simulink model "simulacion_sin_f"  (R2021a)
settings: Solver=VariableStepAuto  StartTime=0.0  StopTime=10.0  RelTol=1e-3
libraries: simulink x1
settings Model: Creator=franc  LastModifiedBy=franc

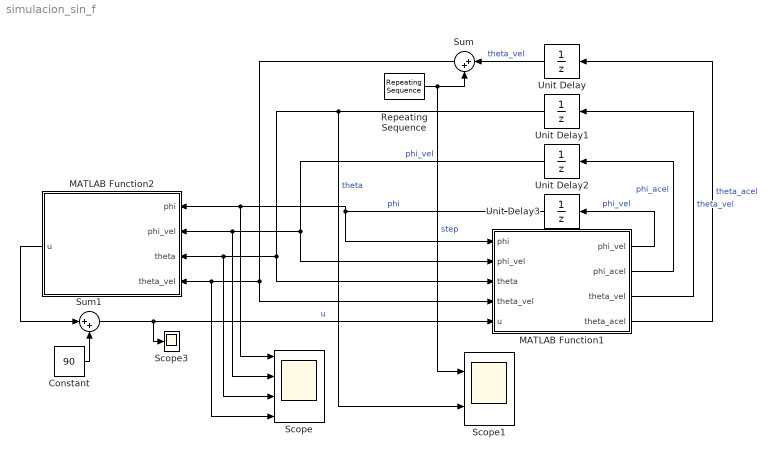
== system simulacion_sin_f ==
  Constant : Constant  Value=90
  MATLAB Function1 : MATLAB Function  TreatAsAtomicUnit=on
  MATLAB Function2 : MATLAB Function  TreatAsAtomicUnit=on
  Repeating Sequence : simulink/Sources/Repeating Sequence  rep_seq_t=[0 0.04 0.045 0.09 0.3 2.045 2.05 2.12 10]  rep_seq_y=[0 0 -10 0 0 0 10 0 0]
  Scope : Scope  NumInputPorts=4
  Scope1 : Scope  NumInputPorts=2
  Scope3 : Scope
  Sum : Sum  Inputs=|++
  Sum1 : Sum  Inputs=|++
  Unit Delay : UnitDelay  SampleTime=0.01  HasFrameUpgradeWarning=on
  Unit Delay1 : UnitDelay  SampleTime=0.01  HasFrameUpgradeWarning=on
  Unit Delay2 : UnitDelay  SampleTime=0.01  HasFrameUpgradeWarning=on
  Unit Delay3 : UnitDelay  InitialCondition=90  SampleTime=0.01  HasFrameUpgradeWarning=on
  wires:
  MATLAB Function1/1(phi_vel) -> Unit Delay3/1  "phi_vel"
  MATLAB Function1/2(phi_acel) -> Unit Delay2/1  "phi_acel"
  Unit Delay2/1 -> MATLAB Function2/2(phi_vel), Scope/2, MATLAB Function1/2("phi_vel ")  "phi_vel"
  MATLAB Function1/3(theta_vel) -> Unit Delay1/1  "theta_vel"
  MATLAB Function1/4(theta_acel) -> Unit Delay/1  "theta_acel"
  Unit Delay3/1 -> Scope/1, MATLAB Function2/1(phi), MATLAB Function1/1(phi)  "phi"
  Unit Delay1/1 -> Scope1/2, MATLAB Function2/3(theta), Scope/3, MATLAB Function1/3(theta)  "theta"
  MATLAB Function2/1(u) -> Sum1/1
  Sum1/1 -> Scope3/1, MATLAB Function1/5(u)  "u"
  Constant/1 -> Sum1/2
  Unit Delay/1 -> Sum/1  "theta_vel"
  Repeating Sequence/1 -> Sum/2, Scope1/1  "step"
  Sum/1 -> MATLAB Function1/4("theta_vel "), Scope/4, MATLAB Function2/4(theta_vel)

== matlab function simulacion_sin_f/MATLAB Function1 ==
  data: phi input; phi_vel input; theta input; theta_vel input; u input; phi_vel output; phi_acel output; theta_vel output; theta_acel output
function [phi_vel,phi_acel,theta_vel,theta_acel] = fcn(phi,phi_vel,theta,theta_vel,u)

Ad = [
    1.0000    0.0100         0         0;
   -0.5765    0.9895   -2.1322   -0.2132;
         0         0    1.0000    0.0100;
         0         0   -2.5000    0.7500;
];
   
Bd = [
         0;
  2.132250;
         0;
  2.500000
];

x  = [theta theta_vel phi phi_vel];
x_dot = Ad * x' + Bd * u;
theta_vel = x_dot(1);
theta_acel = x_dot(2);
phi_vel = x_dot(3);
phi_acel = x_dot(4);

== matlab function simulacion_sin_f/MATLAB Function2 ==
  data: phi input; phi_vel input; theta input; theta_vel input; u output
function u = fcn(phi,phi_vel,theta,theta_vel)
    K = [-0.5, 0.001, 0.7, -0.005];
    u = K(1) * theta + K(2) * theta_vel + K(3) * (phi - 90) + K(4) * phi_vel;
